simulink model "tune2"  (R2018a)
settings: Solver=FixedStepAuto  StartTime=0.0  StopTime=3.5  FixedStep=0.02  RelTol=1e-3  EnableMultiTasking=on
undefined symbols (not defined in the file or in its folder): DiscIntNeverNeededParam
libraries: simulink_extras x4, simulink x2
settings Model: ExtModeTrigDuration=2  Creator=JOEYUCHECKED  LastModifiedBy=rahul
settings OptimizationCC: EnhancedBackFolding=on  PassReuseOutputArgsAs=Individual arguments  MaxStackSize=64  OptimizeBlockOrder=speed  DifferentSizesBufferReuse=on
settings DebuggingCC: ParameterTunabilityLossMsg=error
settings HardwareCC: ProdBitPerInt=16  ProdBitPerPointer=16  ProdBitPerSizeT=16  ProdBitPerPtrDiffT=16  ProdLargestAtomicFloat=None  ProdWordSize=8  ProdHWDeviceType=Atmel->AVR
settings SFSimCC: MATLABDynamicMemAlloc=off
settings RTWCC: SystemTargetFile=ert.tlc  HardwareBoard=Arduino Uno  TLCOptions=-aInlineSetEventsForThisBaseRateFcn=TLC_FALSE -aSuppressMultiTaskScheduler=TLC_FALSE -aRateBasedStepFcn=1  TemplateMakefile=ert_default_tmf  GenerateReport=on  Toolchain=Arduino AVR  BuildConfiguration=Faster Runs  IncludeHyperlinkInReport=on  LaunchReport=on  GenerateTraceInfo=on  GenerateTraceReport=on  GenerateTraceReportSl=on  GenerateTraceReportSf=on  GenerateTraceReportEml=on
settings CodeAppCC: ForceParamTrailComments=on  IgnoreCustomStorageClasses=off  OperatorAnnotations=on  SimulinkDataObjDesc=on  SFDataObjDesc=on  InsertBlockDesc=on
settings ERTTargetCC: SupportContinuousTime=on  SupportVariableSizeSignals=on

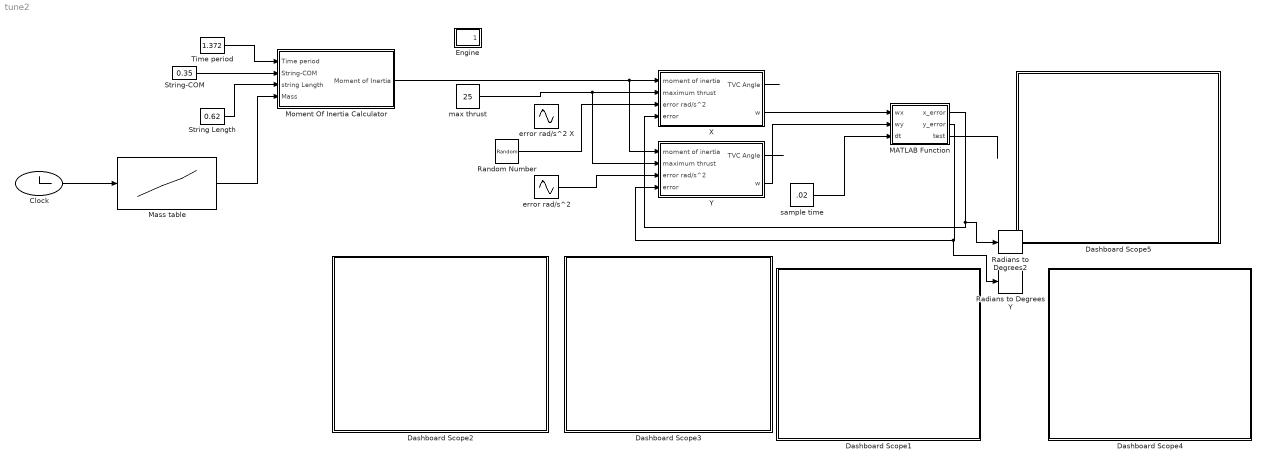
== system tune2 ==
  Clock : Clock
  Dashboard Scope1 : Subsystem  DialogController=hmiCreateDDGDialog  IsWebBlock=on  mask(MWDashboardBlock){webBlockId=79388a0e-acf4-4a0f-9f6d-7a65b6fe74ae, webBlockType=sdiscope, ShowInitialText=on, HMISrcModelName=tune2}
      mask prompts: webBlockId "WebBlock Id"; webBlockType "WebBlock Type"; HMISrcModelName "Source Model"
      mask help: SimulinkHMI:dialogs:HMIScopeDialogDesc
      mask Help: helpview([docroot '/mapfiles/simulink.map'], 'hmi_scope')
      mask Display:
      | if strcmp(get_param(bdroot(gcb),'BlockDiagramType'), 'library')
      |     image([(matlabroot) '/toolbox/simulink/hmi/icons/DashboardScope.png']);
      | end
  Dashboard Scope2 : Subsystem  DialogController=hmiCreateDDGDialog  IsWebBlock=on  mask(MWDashboardBlock){webBlockId=90f90a36-db43-40ab-b237-b326ceb92136, webBlockType=sdiscope, ShowInitialText=on, HMISrcModelName=tune2}
      mask prompts: webBlockId "WebBlock Id"; webBlockType "WebBlock Type"; HMISrcModelName "Source Model"
      mask help: SimulinkHMI:dialogs:HMIScopeDialogDesc
      mask Help: helpview([docroot '/mapfiles/simulink.map'], 'hmi_scope')
      mask Display:
      | if strcmp(get_param(bdroot(gcb),'BlockDiagramType'), 'library')
      |     image([(matlabroot) '/toolbox/simulink/hmi/icons/DashboardScope.png']);
      | end
  Dashboard Scope3 : Subsystem  DialogController=hmiCreateDDGDialog  IsWebBlock=on  mask(MWDashboardBlock){webBlockId=200297c4-bc4f-4d0c-b2fb-30ef607173bc, webBlockType=sdiscope, ShowInitialText=on, HMISrcModelName=tune2}
      mask prompts: webBlockId "WebBlock Id"; webBlockType "WebBlock Type"; HMISrcModelName "Source Model"
      mask help: SimulinkHMI:dialogs:HMIScopeDialogDesc
      mask Help: helpview([docroot '/mapfiles/simulink.map'], 'hmi_scope')
      mask Display:
      | if strcmp(get_param(bdroot(gcb),'BlockDiagramType'), 'library')
      |     image([(matlabroot) '/toolbox/simulink/hmi/icons/DashboardScope.png']);
      | end
  Dashboard Scope4 : Subsystem  DialogController=hmiCreateDDGDialog  IsWebBlock=on  mask(MWDashboardBlock){webBlockId=39e51e81-36ff-42c4-bd8e-4409406b6c93, webBlockType=sdiscope, ShowInitialText=on, HMISrcModelName=tune2}
      mask prompts: webBlockId "WebBlock Id"; webBlockType "WebBlock Type"; HMISrcModelName "Source Model"
      mask help: SimulinkHMI:dialogs:HMIScopeDialogDesc
      mask Help: helpview([docroot '/mapfiles/simulink.map'], 'hmi_scope')
      mask Display:
      | if strcmp(get_param(bdroot(gcb),'BlockDiagramType'), 'library')
      |     image([(matlabroot) '/toolbox/simulink/hmi/icons/DashboardScope.png']);
      | end
  Dashboard Scope5 : Subsystem  DialogController=hmiCreateDDGDialog  IsWebBlock=on  mask(MWDashboardBlock){webBlockId=c88cf3d1-9880-470f-8eff-1f6e97b7395e, webBlockType=sdiscope, ShowInitialText=on, HMISrcModelName=tune2}
      mask prompts: webBlockId "WebBlock Id"; webBlockType "WebBlock Type"; HMISrcModelName "Source Model"
      mask help: SimulinkHMI:dialogs:HMIScopeDialogDesc
      mask Help: helpview([docroot '/mapfiles/simulink.map'], 'hmi_scope')
      mask Display:
      | if strcmp(get_param(bdroot(gcb),'BlockDiagramType'), 'library')
      |     image([(matlabroot) '/toolbox/simulink/hmi/icons/DashboardScope.png']);
      | end
  Engine : Subsystem
  MATLAB Function : MATLAB Function  TreatAsAtomicUnit=on
  Mass table : Lookup  InputValues=[0,1]  Table=[0.975,.8]  LookUpMeth=Use Input Nearest  SaturateOnIntegerOverflow=on
  Moment Of Inertia Calculator : Subsystem
  Radians to Degrees Y : simulink_extras/Transformations/Radians to Degrees
  Radians to Degrees2 : simulink_extras/Transformations/Radians to Degrees
  Random Number : RandomNumber  Mean=1  Variance=.2  SampleTime=.02
  String Length : Constant  Value=0.62
  String-COM : Constant  Value=0.35
  Time period : Constant  Value=1.372
  X : Subsystem
  Y : Subsystem
  error rad/s^2 : Sin  Amplitude=pi  Frequency=4  SampleTime=0
  error rad/s^2 X : Sin  Amplitude=pi  SampleTime=0
  max thrust : Constant  Value=25
  sample time : Constant  Value=.02
  wires:
  max thrust/1 -> X/2(maximum thrust), Y/2(maximum thrust)
  String-COM/1 -> Moment Of Inertia Calculator/2(String-COM)
  Time period/1 -> Moment Of Inertia Calculator/1(Time period)
  Moment Of Inertia Calculator/1(Moment of Inertia) -> X/1(moment of inertia), Y/1(moment of inertia)
  String Length/1 -> Moment Of Inertia Calculator/3(string Length)
  Mass table/1 -> Moment Of Inertia Calculator/4(Mass)
  Clock/1 -> Mass table/1
  MATLAB Function/1(x_error) -> Radians to Degrees2/1, X/4(error)
  MATLAB Function/2(y_error) -> Radians to Degrees Y/1, Y/4(error)
  sample time/1 -> MATLAB Function/3(dt)
  X/2(w) -> MATLAB Function/1(wx)
  Y/2(w) -> MATLAB Function/2(wy)
  Y/1(TVC Angle) -> ?
  MATLAB Function/3(test) -> ?
  error rad/s^2/1 -> Y/3(error rad/s^2)
  X/1(TVC Angle) -> ?
  Random Number/1 -> X/3(error rad/s^2)

== system tune2/Dashboard Scope1 ==

== system tune2/Dashboard Scope2 ==

== system tune2/Dashboard Scope3 ==

== system tune2/Dashboard Scope4 ==

== system tune2/Dashboard Scope5 ==

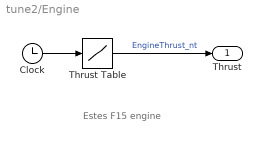
== system tune2/Engine ==
  note: Estes F15 engine
  Clock : Clock
  Thrust Table : Lookup  InputValues=|  Table=[0,12.5,25,16.5,15.25,15,14.5,14.5,14.25,14,13,13,0]  LookUpMeth=Interpolation-Use End Values  SaturateOnIntegerOverflow=on
      | [0,
      | 0.25,
      | 0.5,
      | 0.75,
      | 1,
      | 1.25,
      | 1.5,
      | 2,
      | 2.25,
      | 2.5,
      | 3,
      | 3.25,
      | 3.5]
  Thrust : Outport
  wires:
  Clock/1 -> Thrust Table/1
  Thrust Table/1 -> Thrust/1  "EngineThrust_nt"

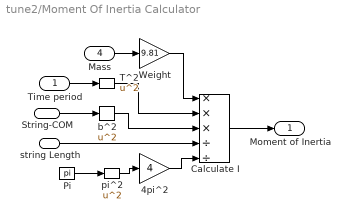
== system tune2/Moment Of Inertia Calculator ==
  Time period : Inport
  String-COM : Inport  Port=2
  string Length : Inport  Port=3
  Mass : Inport  Port=4
  4pi^2 : Gain  Gain=4
  Calculate I : Product  Inputs=***//
  Pi : Constant  Value=pi
  T^2 : Math  Operator=square  SaturateOnIntegerOverflow=on
  Weight : Gain  Gain=9.81
  b^2 : Math  Operator=square  SaturateOnIntegerOverflow=on
  pi^2 : Math  Operator=square  SaturateOnIntegerOverflow=on
  Moment of Inertia : Outport
  wires:
  Time period/1 -> T^2/1
  Calculate I/1 -> Moment of Inertia/1
  string Length/1 -> Calculate I/4
  Mass/1 -> Weight/1
  Weight/1 -> Calculate I/1
  pi^2/1 -> 4pi^2/1
  b^2/1 -> Calculate I/3
  T^2/1 -> Calculate I/2
  String-COM/1 -> b^2/1
  Pi/1 -> pi^2/1
  4pi^2/1 -> Calculate I/5

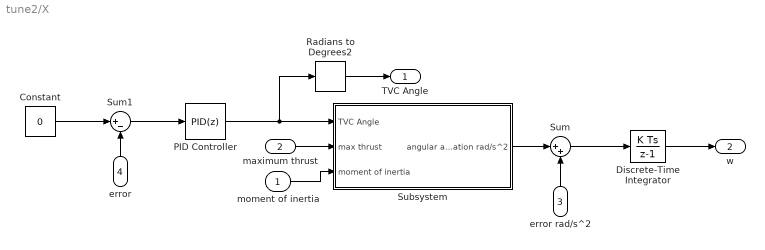
== system tune2/X ==
  moment of inertia : Inport
  maximum thrust : Inport  Port=2
  error rad/s^2 : Inport  Port=3
  error : Inport  Port=4
  Constant : Constant  Value=0
  Discrete-Time Integrator : DiscreteIntegrator  SampleTime=-1  ICPrevOutput=DiscIntNeverNeededParam  ICPrevScaledInput=DiscIntNeverNeededParam
  PID Controller : simulink/Continuous/PID Controller  Controller=PID  TimeDomain=Discrete-time  SampleTime=-1  IntegratorMethod=Forward Euler  FilterMethod=Forward Euler  Form=Parallel  UseFilter=on  ControllerParametersSource=internal  P=57.6314881231161  I=186.197505740408  D=0.347453352722497  N=43.1955233851284  InitialConditionSource=internal  InitialConditionForIntegrator=0  InitialConditionForFilter=0  ExternalReset=none  LimitOutput=off  UpperSaturationLimit=inf  LowerSaturationLimit=-inf  LinearizeAsGain=on  AntiWindupMode=none  Kb=1  TrackingMode=off  Kt=1  PParamMin=[]  PParamMax=[]  IParamMin=[]  IParamMax=[]  DParamMin=[]  DParamMax=[]  NParamMin=[]  NParamMax=[]  KbParamMin=[]  KbParamMax=[]  KtParamMin=[]  KtParamMax=[]  POutMin=[]  POutMax=[]  IOutMin=[]  IOutMax=[]  DOutMin=[]  DOutMax=[]  NOutMin=[]  NOutMax=[]  KbOutMin=[]  KbOutMax=[]  KtOutMin=[]  KtOutMax=[]  IntegratorOutMin=[]  IntegratorOutMax=[]  FilterOutMin=[]  FilterOutMax=[]  SumOutMin=[]  SumOutMax=[]  SumI1OutMin=[]  SumI1OutMax=[]  SumI2OutMin=[]  SumI2OutMax=[]  SumI3OutMin=[]  SumI3OutMax=[]  SumDOutMin=[]  SumDOutMax=[]  SaturationOutMin=[]  SaturationOutMax=[]  IntegratorContinuousStateAttributes=''  IntegratorStateMustResolveToSignalObject=off  IntegratorRTWStateStorageClass=Auto  FilterContinuousStateAttributes=''  FilterStateMustResolveToSignalObject=off  FilterRTWStateStorageClass=Auto  DifferentiatorICPrevScaledInput=0  DifferentiatorOutMin=[]  DifferentiatorOutMax=[]  FilterDiffOutCoefMin=[]  FilterDiffOutCoefMax=[]  SumDenOutMin=[]  SumDenOutMax=[]  SumNumOutMin=[]  SumNumOutMax=[]  ReciprocalOutMin=[]  ReciprocalOutMax=[]  DivideOutMin=[]  DivideOutMax=[]  TunerSelectOption=Transfer Function Based (PID Tuner App)
  Radians to Degrees2 : simulink_extras/Transformations/Radians to Degrees
  Subsystem : Subsystem
  Sum : Sum  Inputs=|++
  Sum1 : Sum  Inputs=|+-
  TVC Angle : Outport
  w : Outport  Port=2
  wires:
  moment of inertia/1 -> Subsystem/3(moment of inertia)
  maximum thrust/1 -> Subsystem/2(max thrust)
  Sum/1 -> Discrete-Time Integrator/1
  Constant/1 -> Sum1/1
  Subsystem/1(angular acceleration rad/s^2) -> Sum/1
  Radians to Degrees2/1 -> TVC Angle/1
  error rad/s^2/1 -> Sum/2
  Discrete-Time Integrator/1 -> w/1
  error/1 -> Sum1/2
  Sum1/1 -> PID Controller/1
  PID Controller/1 -> Radians to Degrees2/1, Subsystem/1(TVC Angle)

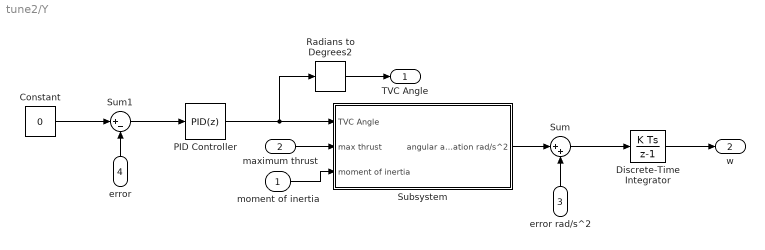
== system tune2/Y ==
  moment of inertia : Inport
  maximum thrust : Inport  Port=2
  error rad/s^2 : Inport  Port=3
  error : Inport  Port=4
  Constant : Constant  Value=0
  Discrete-Time Integrator : DiscreteIntegrator  SampleTime=-1  ICPrevOutput=DiscIntNeverNeededParam  ICPrevScaledInput=DiscIntNeverNeededParam
  PID Controller : simulink/Continuous/PID Controller  Controller=PID  TimeDomain=Discrete-time  SampleTime=-1  IntegratorMethod=Forward Euler  FilterMethod=Forward Euler  Form=Parallel  UseFilter=on  ControllerParametersSource=internal  P=57.6314881231161  I=186.197505740408  D=0.347453352722497  N=43.1955233851284  InitialConditionSource=internal  InitialConditionForIntegrator=0  InitialConditionForFilter=0  ExternalReset=none  LimitOutput=off  UpperSaturationLimit=inf  LowerSaturationLimit=-inf  LinearizeAsGain=on  AntiWindupMode=none  Kb=1  TrackingMode=off  Kt=1  PParamMin=[]  PParamMax=[]  IParamMin=[]  IParamMax=[]  DParamMin=[]  DParamMax=[]  NParamMin=[]  NParamMax=[]  KbParamMin=[]  KbParamMax=[]  KtParamMin=[]  KtParamMax=[]  POutMin=[]  POutMax=[]  IOutMin=[]  IOutMax=[]  DOutMin=[]  DOutMax=[]  NOutMin=[]  NOutMax=[]  KbOutMin=[]  KbOutMax=[]  KtOutMin=[]  KtOutMax=[]  IntegratorOutMin=[]  IntegratorOutMax=[]  FilterOutMin=[]  FilterOutMax=[]  SumOutMin=[]  SumOutMax=[]  SumI1OutMin=[]  SumI1OutMax=[]  SumI2OutMin=[]  SumI2OutMax=[]  SumI3OutMin=[]  SumI3OutMax=[]  SumDOutMin=[]  SumDOutMax=[]  SaturationOutMin=[]  SaturationOutMax=[]  IntegratorContinuousStateAttributes=''  IntegratorStateMustResolveToSignalObject=off  IntegratorRTWStateStorageClass=Auto  FilterContinuousStateAttributes=''  FilterStateMustResolveToSignalObject=off  FilterRTWStateStorageClass=Auto  DifferentiatorICPrevScaledInput=0  DifferentiatorOutMin=[]  DifferentiatorOutMax=[]  FilterDiffOutCoefMin=[]  FilterDiffOutCoefMax=[]  SumDenOutMin=[]  SumDenOutMax=[]  SumNumOutMin=[]  SumNumOutMax=[]  ReciprocalOutMin=[]  ReciprocalOutMax=[]  DivideOutMin=[]  DivideOutMax=[]  TunerSelectOption=Transfer Function Based (PID Tuner App)
  Radians to Degrees2 : simulink_extras/Transformations/Radians to Degrees
  Subsystem : Subsystem
  Sum : Sum  Inputs=|++
  Sum1 : Sum  Inputs=|+-
  TVC Angle : Outport
  w : Outport  Port=2
  wires:
  moment of inertia/1 -> Subsystem/3(moment of inertia)
  maximum thrust/1 -> Subsystem/2(max thrust)
  Sum/1 -> Discrete-Time Integrator/1
  Constant/1 -> Sum1/1
  Subsystem/1(angular acceleration rad/s^2) -> Sum/1
  Radians to Degrees2/1 -> TVC Angle/1
  error rad/s^2/1 -> Sum/2
  Discrete-Time Integrator/1 -> w/1
  error/1 -> Sum1/2
  Sum1/1 -> PID Controller/1
  PID Controller/1 -> Radians to Degrees2/1, Subsystem/1(TVC Angle)

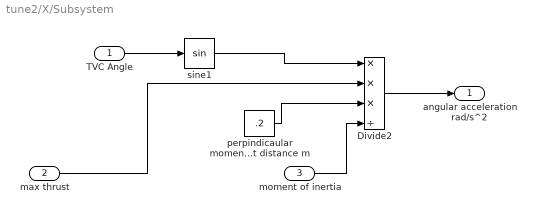
== system tune2/X/Subsystem ==
  TVC Angle : Inport
  max thrust : Inport  Port=2
  moment of inertia : Inport  Port=3
  Divide2 : Product  Inputs=***/
  perpindicaular moment distance m : Constant  Value=.2
  sine1 : Trigonometry
  angular acceleration rad/s^2 : Outport
  wires:
  max thrust/1 -> Divide2/2
  sine1/1 -> Divide2/1
  perpindicaular moment distance m/1 -> Divide2/3
  moment of inertia/1 -> Divide2/4
  TVC Angle/1 -> sine1/1
  Divide2/1 -> angular acceleration rad/s^2/1

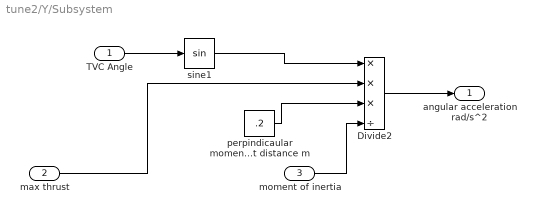
== system tune2/Y/Subsystem ==
  TVC Angle : Inport
  max thrust : Inport  Port=2
  moment of inertia : Inport  Port=3
  Divide2 : Product  Inputs=***/
  perpindicaular moment distance m : Constant  Value=.2
  sine1 : Trigonometry
  angular acceleration rad/s^2 : Outport
  wires:
  max thrust/1 -> Divide2/2
  sine1/1 -> Divide2/1
  perpindicaular moment distance m/1 -> Divide2/3
  moment of inertia/1 -> Divide2/4
  TVC Angle/1 -> sine1/1
  Divide2/1 -> angular acceleration rad/s^2/1

== matlab function tune2/MATLAB Function ==
  settings: updateMethod=DISCRETE
  data: wx input; wy input; x_error output; y_error output; dt input; test output
function [x_error, y_error, test] = fcn(wx, wy, dt)

persistent q_orientation;

if isempty(q_orientation)
    q_orientation = [1 0 0 0];
end

w = [wy wx 0];
angle = norm(w) * dt/2;

if eq(w, [0 0 0])
    axis_angle_of_rotation = [0 0 0 0];
else
    axis_angle_of_rotation = [angle w/norm(w)];
end

quaternion_axis_angle_of_rotation = [cos(angle) sin(angle)*axis_angle_of_rotation(2:4)];

q_orientation = quatnormalize(quatmultiply(q_orientation, quaternion_axis_angle_of_rotation));

if q_orientation(1) < 0
    q_orientation = -q_orientation;
end

test = q_orientation;
if abs(q_orientation(1)) ~= 1 %is it rotated 0 degrees
    s = sin(acos(q_orientation(1)));
    angle_axis_orientation = [2*acos(q_orientation(1)) q_orientation(2:4)/s];
    y_error = angle_axis_orientation(1) * angle_axis_orientation(2);
    x_error = angle_axis_orientation(1) * angle_axis_orientation(3);
else 
    y_error = 0;
    x_error = 0;
end
